simulink model "example_autopilot"  (R2022b)
settings: Solver=VariableStepAuto  StartTime=0.0  StopTime=10.0  RelTol=1e-3
settings Model: DataDictionary=uorb_msg.sldd  Creator=zhanfuyu  LastModifiedBy=zhanfuyu

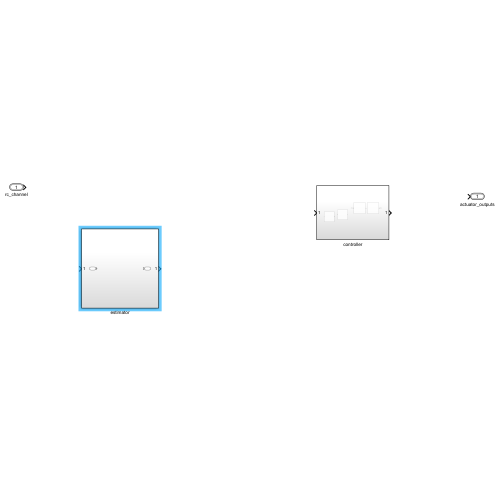
[thumbnail: Simulink's stored preview of the top-level diagram]
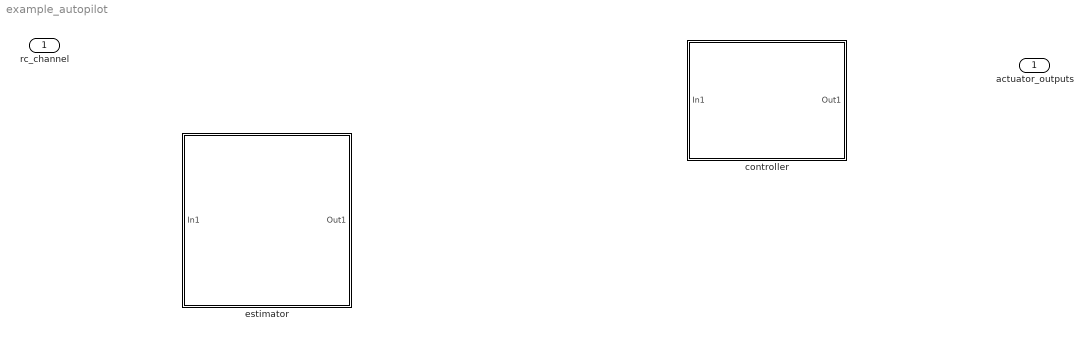
== system example_autopilot ==
  rc_channel : Inport  OutDataTypeStr=Bus: rc_channels_s
  controller : Subsystem
  estimator : Subsystem
  actuator_outputs : Outport  OutDataTypeStr=Bus: actuator_outputs_s

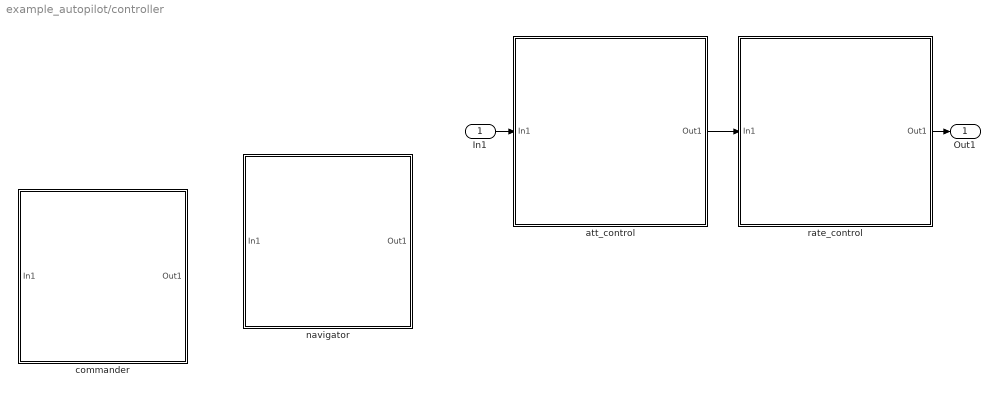
== system example_autopilot/controller ==
  In1 : Inport
  att_control : Subsystem
  commander : Subsystem
  navigator : Subsystem
  rate_control : Subsystem
  Out1 : Outport
  wires:
  att_control/1(Out1) -> rate_control/1(In1)
  In1/1 -> att_control/1(In1)
  rate_control/1(Out1) -> Out1/1

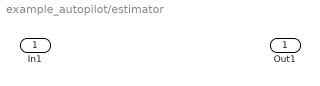
== system example_autopilot/estimator ==
  In1 : Inport
  Out1 : Outport

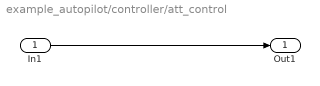
== system example_autopilot/controller/att_control ==
  In1 : Inport
  Out1 : Outport
  wires:
  In1/1 -> Out1/1

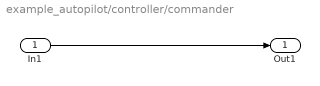
== system example_autopilot/controller/commander ==
  In1 : Inport
  Out1 : Outport
  wires:
  In1/1 -> Out1/1

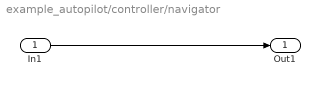
== system example_autopilot/controller/navigator ==
  In1 : Inport
  Out1 : Outport
  wires:
  In1/1 -> Out1/1

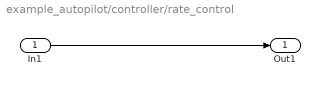
== system example_autopilot/controller/rate_control ==
  In1 : Inport
  Out1 : Outport
  wires:
  In1/1 -> Out1/1
